simulink model "TRIAD"  (R2017a)
settings: Solver=ode4  StartTime=0.0  StopTime=20000  FixedStep=0.1  RelTol=1e-3  EnableMultiTasking=on
undefined symbols (not defined in the file): mbaseserialmask, RxBuffer
libraries: xpcseriallib x17, vrlib x7, slrtlib x4, sharedtransform x3, sharedutil x2, dspinverses x2, dspmathops x2, simulink x1, dspsigops x1
(part 1 of 3)
settings Model: Creator=yhj  LastModifiedBy=ATLAS
settings SolverCC: EnableConcurrentExecution=on  ConcurrentTasks=on  AutoInsertRateTranBlk=on
settings DataIOCC: SaveFormat=StructureWithTime
settings OptimizationCC: BlockReduction=off  OptimizeBlockIOStorage=off  BufferReuse=off  GlobalBufferReuse=off  ExpressionFolding=off  LocalBlockOutputs=off
settings HardwareCC: ProdBitPerPointer=32  ProdBitPerSizeT=32  ProdBitPerPtrDiffT=32  ProdLargestAtomicFloat=None  ProdWordSize=32  ProdLongLongMode=on  ProdHWDeviceType=Generic->32-bit x86 compatible
settings RTWCC: SystemTargetFile=slrt.tlc  TemplateMakefile=slrt_default_tmf  Description=Simulink Real-Time  RTWCompilerOptimization=on
settings SimulinkRealTimeCC: xPCConcurrentTasks=on

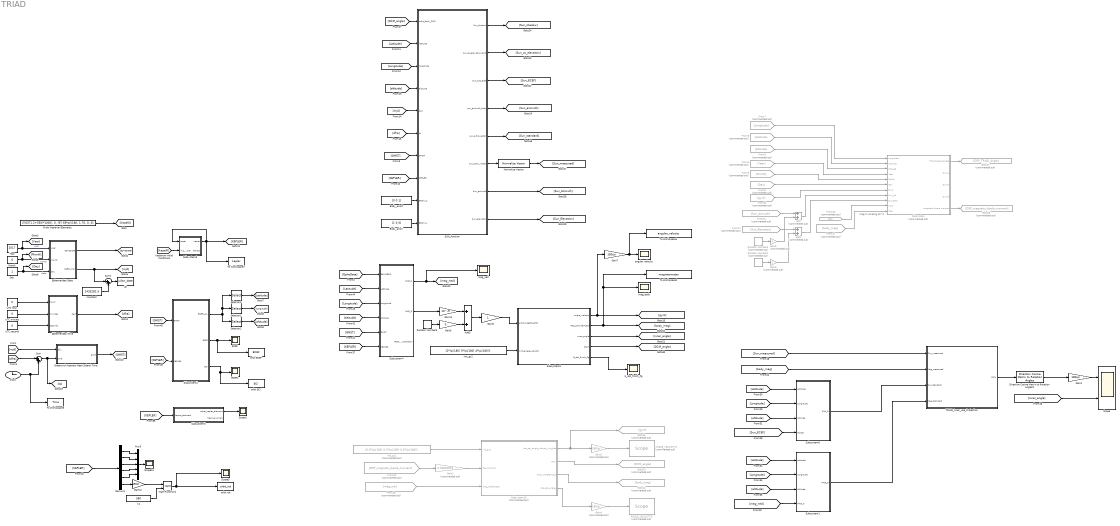
== system TRIAD ==
  note: mag =>scaling 10^3
  ANGLE_VELOCITY2 : slrtlib/Displays and Logging/Scope   Commented=on  scopeno=3  scopetype=Target  autostart=on  viewmode=Numerical  formatstr='%15.6f'  grid=on  ylimits=[-180,180]  nosamples=3  noprepostsamples=0  interleave=10  triggermode=FreeRun  triggersignal=1  trigsignalfromport=off  triggerlevel=0.0  triggerslope=Either  triggerscope=1  triggersample=0  filename=ANGLE2.dat  mode=Lazy  writesize=512  autorestart=off  dynamicfilemode=off  maxwritefilesize=512*1024^2
  ANGLE_VELOCITY3 : slrtlib/Displays and Logging/Scope   Commented=on  scopeno=7  scopetype=Target  autostart=on  viewmode=Numerical  formatstr='%15.6f'  grid=on  ylimits=[-180,180]  nosamples=3  noprepostsamples=0  interleave=10  triggermode=FreeRun  triggersignal=1  trigsignalfromport=off  triggerlevel=0.0  triggerslope=Either  triggerscope=1  triggersample=0  filename=ANGLE2.dat  mode=Lazy  writesize=512  autorestart=off  dynamicfilemode=off  maxwritefilesize=512*1024^2
  Add3 : Sum
  Body_axisX : Constant  Value=[1 0 0]  VectorParams1D=off
  Body_axisZ : Constant  Value=[0 0 1]  VectorParams1D=off
  Clock : Clock
  Day : Constant
  Demux3 : Demux  Outputs=6
  Direction Cosine Matrix to Rotation Angles2 : sharedtransform/Direction Cosine Matrix to Rotation Angles  rotationOrder=ZYX  lim=Default
  ECEF : Scope
  ECEF1 : Scope
  Ephemerides Date : Subsystem
  Ephemerides Time : MATLAB Function  TreatAsAtomicUnit=on
  From17 : From  Commented=on  GotoTag=Sun_Elevation
  From19 : From  Commented=on  GotoTag=mag_orb
  From20 : From  Commented=on  GotoTag=DSP_magnetic_dipole_moment
  From21 : From  Commented=on  GotoTag=gyro
  From23 : From  Commented=on  GotoTag=ts
  From4 : From  Commented=on  GotoTag=Year
  From47 : From  Commented=on  GotoTag=body_mag
  From5 : From  Commented=on  GotoTag=Month
  From51 : From  Commented=on  GotoTag=Sun_Azimuth
  From6 : From  Commented=on  GotoTag=Day
  From7 : From  Commented=on  GotoTag=Longitude
  From8 : From  Commented=on  GotoTag=Latitude
  From9 : From  Commented=on  GotoTag=altitude
  Gain1 : Gain  Gain=180/pi
  Gain11 : Gain  Gain=10^-9
  Gain12 : Gain  Gain=180/pi
  Gain2 : Gain  Commented=on  Gain=0.00000001
  Gain3 : Gain  Commented=on  Gain=180/pi
  Gain4 : Gain  Commented=on  Gain=180/pi
  Gain5 : Gain  Gain=0
  Gain6 : Gain
  Gain7 : Gain  Gain=180/pi
  Gain8 : Gain  Commented=on  Gain=0
  Gain9 : Gain  Commented=on  Gain=0
  Goto12 : Goto  Commented=on  GotoTag=body_mag
  Goto23 : Goto  Commented=on  GotoTag=DCM_angle
  Goto25 : Goto  Commented=on  GotoTag=gyro
  Goto26 : Goto  Commented=on  GotoTag=DSP_magnetic_dipole_moment
  Goto27 : Goto  Commented=on  GotoTag=DSP_TRIAD_Angle
  Greenwich Aparent Mean Sideral Time : MATLAB Function  TreatAsAtomicUnit=on
  JD : ToWorkspace  VariableName=Julian_date  SampleTime=-1
  Math Function1 : Math  Operator=rem  SaturateOnIntegerOverflow=on
  Month : Constant  Value=6
  Mux3 : Mux  Inputs=5
  Normalize Vector : vrlib/Utilities/Normalize Vector  maxzero=0
      settings: SourceProductName=Simulink 3D Animation  SourceProductBaseCode=VR
  Orbit Keplerian Elements : Constant  Value=[((6371.2+550)*1000), 0, (97.69*pi)/180, 1.76, 0, 0]
  Random Number2 : RandomNumber  Commented=on  Variance=0.035^2
  Random Number3 : RandomNumber  Commented=on  Variance=0.035^2
  Random Number9 : RandomNumber  Variance=(3*10^-7)^2
  SUN_function : Subsystem
  Scope : Scope  NumInputPorts=2
  Scope1 : Scope
  Scope24 : Scope
  Scope3 : Scope
  Selector1 : Selector  InputPortWidth=3  IndexOptions=Index vector (dialog)  Indices=[1]  OutputSizes=1
  Selector2 : Selector  InputPortWidth=3  IndexOptions=Index vector (dialog)  Indices=[3]  OutputSizes=1
  Selector3 : Selector  InputPortWidth=3  IndexOptions=Index vector (dialog)  Indices=[2]  OutputSizes=1
  Subsystem : Subsystem  Commented=on
  Subsystem1 : Subsystem
  Subsystem10 : Subsystem  Commented=on
  Subsystem2 : Subsystem
  Subsystem3 : Subsystem
  Subsystem4 : Subsystem
  Subsystem5 : Subsystem
  Subsystem6 : Subsystem
  Subsystem9 : Subsystem
  Sum : Sum  Inputs=|++
  Sum1 : Sum  Inputs=|++
  TRIAD_inner_use_Projection : Subsystem
  To Workspace1 : ToWorkspace  VariableName=angular_velocity  SampleTime=-1
  To Workspace2 : ToWorkspace  VariableName=magnetometer  SampleTime=-1
  To Workspace3 : ToWorkspace  VariableName=Time  SampleTime=-1
  To Workspace7 : ToWorkspace  VariableName=kepler  SampleTime=-1
      settings: Save2DSignal=2-D array (concatenate along first dimension)
  UTC hour : Constant  Value=0
  UTC minute : Constant  Value=0
  UTC second : Constant  Value=0
  Year : Constant  Value=2017
  add : Sum  Commented=on
  add1 : Sum  Commented=on
  angular velocity : Scope
  b_dot_finish_flg : Scope
  constant : Constant  Value=2433282.5
  init_gy1 : Constant  Commented=on  Value=[0.5*(pi/180) 0.5*(pi/180) 0.5*(pi/180)]'
  init_gy2 : Constant  Value=[2*(pi/180) 5*(pi/180) 4*(pi/180)]'
  k1 : Constant  Value=360
  mag_body : Scope
  mag_ned : Scope
  orbit ECEF : ToWorkspace  VariableName=ECEF  SampleTime=-1
      settings: Save2DSignal=2-D array (concatenate along first dimension)
  orbit ECI : ToWorkspace  VariableName=ECI  SampleTime=-1
      settings: Save2DSignal=2-D array (concatenate along first dimension)
  orbit rot : ToWorkspace  VariableName=orbit_rot  SampleTime=-1
  wires:
  Gain6/1 -> Subsystem9/1(orbit_mag[GAUSS])
  Subsystem9/1(angle_velocity) -> Gain7/1, [gyro]
  Subsystem10/3(body_mag[GAUSS]) -> Goto12/1
  Subsystem10/2(dcm) -> Goto23/1
  Subsystem9/3(inner_angle) -> [inner_angle]
  SUN_function/8(Sun_elevation) -> [Sun_Elevation]
  SUN_function/1(Sun_shadow) -> [Sun_shadow]
  SUN_function/2(sun_co_elevation_body) -> [Sun_co_elevation]
  UTC minute/1 -> Ephemerides Time/2(minutes)
  Subsystem/5(magnetic dipole moment) -> Goto26/1
  [KEPLER] -> Subsystem2/2(KEPLER)
  From47/1 -> Subsystem/11(Mag)
  Subsystem6/1(SUN_O) -> TRIAD_inner_use_Projection/3(Sun_standard)
  [KEPLER] -> Subsystem4/6(KEPLER)
  SUN_function/7(Sun_azimuth) -> [Sun_Azimuth]
  Subsystem3/1(other_kepler_element) -> Scope1/1
  [dfra] -> Sum/1
  Ephemerides Time/1(dayf) -> [dfra]
  Selector1/1 -> [Longitude]
  Greenwich Aparent Mean Sideral Time/1(gwst) -> [GMST]
  UTC second/1 -> Ephemerides Time/3(seconds)
  Day/1 -> [Day], Ephemerides Date/3(day)  "date"
  [KEPLER] -> SUN_function/8(KEPLER)
  Selector3/1 -> [Latitude]
  From7/1 -> Subsystem/1(Longitude)
  Sum/1 -> [ts], Greenwich Aparent Mean Sideral Time/2(time)
  Ephemerides Date/2(CNES_mdj) -> Sum1/1, [mjd]
  [Longitude] -> Subsystem6/2(Longitude)
  Sum1/1 -> JD/1
  Year/1 -> Ephemerides Date/1(year), [Year]  "year"
  [KEPLER] -> Subsystem3/1(kepler_element)
  Clock/1 -> To Workspace3/1, Sum/2
  UTC hour/1 -> Ephemerides Time/1(hours)
  TRIAD_inner_use_Projection/1(DCM) -> Direction Cosine Matrix to Rotation Angles2/1
  Ephemerides Date/1(EpheDate) -> [EpheDate]
  Orbit Keplerian Elements/1 -> [kepel0]
  SUN_function/4(sun_azimuth_body) -> [Sun_azimuth]
  Normalize Vector/1 -> [Sun_measured]
  [dfra] -> SUN_function/6(ts)
  [altitude] -> Subsystem1/3(Altitude)
  [EpheDate] -> Subsystem4/1(EPHMERIS)
  [mag_ned] -> Subsystem1/4(MAG_N)
  [Sun_ECEF] -> Subsystem6/4(SUN_E)
  Subsystem2/1(ECEF_LLA) -> Selector3/1, Selector1/1, Selector2/1
  [Latitude] -> Subsystem4/2(Latitude)
  [body_mag] -> TRIAD_inner_use_Projection/2(Mag_measured)
  [Longitude] -> Subsystem1/2(Longitude)
  [Longitude] -> SUN_function/3(longitude)
  Add3/1 -> Gain6/1
  Month/1 -> [Month], Ephemerides Date/2(month)  "month"
  From4/1 -> Subsystem/4(Year)
  From5/1 -> Subsystem/5(Month)
  [Latitude] -> Subsystem1/1(Latitude)
  constant/1 -> Sum1/2
  add1/1 -> Subsystem/9(Sun_Elev)
  Subsystem1/1(MAG_O) -> TRIAD_inner_use_Projection/4(Mag_standard)
  Subsystem5/1(kepler) -> To Workspace7/1, [KEPLER], Subsystem5/1(kepel)
  [Latitude] -> Subsystem6/1(Latitude)
  Random Number3/1 -> Gain8/1
  add/1 -> Subsystem/8(Sun_Azi)
  From8/1 -> Subsystem/2(Latitude)
  [GMST] -> Subsystem4/5(GMST)
  [altitude] -> Subsystem4/4(Altitude)
  From23/1 -> Subsystem/10(HMS)
  Gain2/1 -> Subsystem10/2(dsp_moment)
  From21/1 -> Subsystem/7(Gyro)
  SUN_function/3(Sun_pos_ecef) -> [Sun_ECEF]
  init_gy1/1 -> Subsystem10/1(init_gyro)
  From51/1 -> add/1
  Random Number9/1 -> Gain5/1
  Random Number2/1 -> Gain9/1
  Gain3/1 -> ANGLE_VELOCITY2/1
  From9/1 -> Subsystem/3(Altitude)
  Subsystem4/1(MAG_N) -> mag_ned/1, [mag_ned]
  [mjd] -> SUN_function/5(djm)
  [Longitude] -> Subsystem4/3(Longitude)
  [altitude] -> Subsystem6/3(Altitude)
  [Latitude] -> SUN_function/2(latitude)
  SUN_function/6(sun_body_vector) -> Normalize Vector/1
  Gain11/1 -> Add3/1
  [Sun_measured] -> TRIAD_inner_use_Projection/1(Sun_measured)
  [DCM_angle] -> SUN_function/1(orbit_body_DCM)
  [mjd] -> Greenwich Aparent Mean Sideral Time/1(diju)
  Body_axisX/1 -> SUN_function/10(BODY_X)
  Subsystem10/1(dsp_cal_angle_velocity_wrt_bdot) -> Goto25/1, Gain3/1
  Subsystem/1(TRAID_result_angle) -> Goto27/1
  SUN_function/5(sun_orbit_vector) -> [Sun_standard]
  [GMST] -> SUN_function/7(GMST)
  [kepel0] -> Subsystem5/2(init_kepler)
  From6/1 -> Subsystem/6(Day)
  From19/1 -> Subsystem10/3(mag_orb[GAUSS])
  Subsystem4/2(MAG_O) -> Gain11/1
  From17/1 -> add1/1
  From20/1 -> Gain2/1
  [altitude] -> SUN_function/4(altitude)
  Body_axisZ/1 -> SUN_function/9(BODY_Z)
  Selector2/1 -> [altitude]
  [GMST] -> Subsystem2/1(GMST)
  Direction Cosine Matrix to Rotation Angles2/1 -> Gain1/1
  Subsystem10/4(dsp_cal_angle_) -> Gain4/1
  Gain4/1 -> ANGLE_VELOCITY3/1
  Gain5/1 -> Add3/2
  Gain8/1 -> add/2
  Gain9/1 -> add1/2
  init_gy2/1 -> Subsystem9/2(iinit_angle_velocity)
  Subsystem9/4(DCM) -> [DCM_angle]
  Subsystem9/2(Mag_body[GAUSS]) -> mag_body/1, To Workspace2/1, [body_mag]
  Gain1/1 -> Scope/1
  [inner_angle] -> Scope/2
  Gain7/1 -> To Workspace1/1, angular velocity/1
  Demux3/3 -> Mux3/3
  Demux3/1 -> Mux3/1
  Math Function1/1 -> Scope3/1, orbit rot/1
  Mux3/1 -> Scope24/1
  Demux3/4 -> Mux3/4
  Demux3/2 -> Mux3/2
  Demux3/6 -> Gain12/1
  Gain12/1 -> Math Function1/1
  k1/1 -> Math Function1/2
  Demux3/5 -> Mux3/5
  [KEPLER] -> Demux3/1
  Subsystem2/2(ECEF) -> ECEF/1, orbit ECEF/1
  Subsystem2/3(ECI) -> ECEF1/1, orbit ECI/1
  Subsystem9/5(B_dot_finish_flg) -> b_dot_finish_flg/1

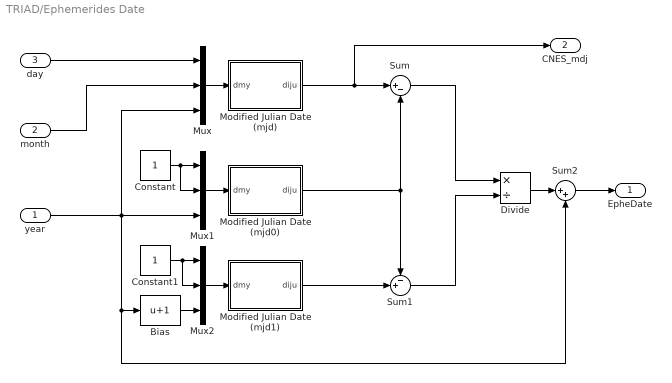
== system TRIAD/Ephemerides Date ==
  year : Inport
  month : Inport  Port=2
  day : Inport  Port=3
  Bias : Bias  Bias=1
  Constant : Constant
  Constant1 : Constant
  Divide : Product  Inputs=*/
  Modified Julian Date (mjd) : MATLAB Function  TreatAsAtomicUnit=on
  Modified Julian Date (mjd0) : MATLAB Function  TreatAsAtomicUnit=on
  Modified Julian Date (mjd1) : MATLAB Function  TreatAsAtomicUnit=on
  Mux : Mux  Inputs=3
  Mux1 : Mux  Inputs=3
  Mux2 : Mux  Inputs=3
  Sum : Sum  Inputs=|+-
  Sum1 : Sum  Inputs=-+|
  Sum2 : Sum  Inputs=|++
  EpheDate : Outport
  CNES_mdj : Outport  Port=2
  wires:
  Sum1/1 -> Divide/2
  Modified Julian Date (mjd1)/1(diju) -> Sum1/2
  month/1 -> Mux/2
  year/1 -> Mux1/3, Mux/3, Bias/1, Sum2/2
  Mux1/1 -> Modified Julian Date (mjd0)/1(dmy)
  day/1 -> Mux/1
  Mux/1 -> Modified Julian Date (mjd)/1(dmy)
  Mux2/1 -> Modified Julian Date (mjd1)/1(dmy)
  Bias/1 -> Mux2/3
  Modified Julian Date (mjd)/1(diju) -> CNES_mdj/1, Sum/1
  Constant1/1 -> Mux2/2, Mux2/1
  Sum/1 -> Divide/1
  Constant/1 -> Mux1/2, Mux1/1
  Modified Julian Date (mjd0)/1(diju) -> Sum1/1, Sum/2
  Divide/1 -> Sum2/1
  Sum2/1 -> EpheDate/1

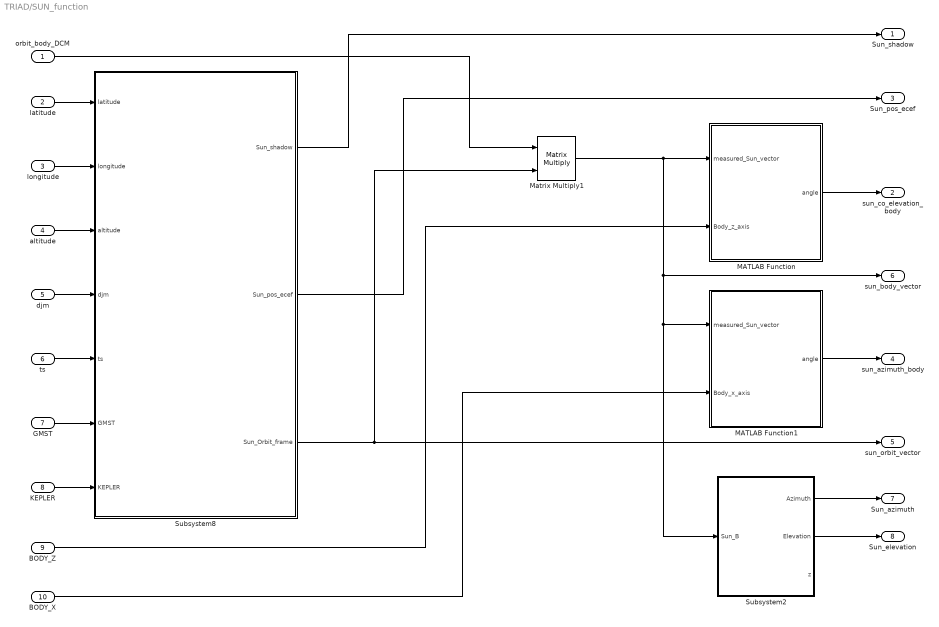
== system TRIAD/SUN_function ==
  orbit_body_DCM : Inport
  latitude : Inport  Port=2
  longitude : Inport  Port=3
  altitude : Inport  Port=4
  djm : Inport  Port=5
  ts : Inport  Port=6
  GMST : Inport  Port=7
  KEPLER : Inport  Port=8
  BODY_Z : Inport  Port=9
  BODY_X : Inport  Port=10
  MATLAB Function : MATLAB Function  TreatAsAtomicUnit=on
  MATLAB Function1 : MATLAB Function  TreatAsAtomicUnit=on
  Matrix Multiply1 : Product  Multiplication=Matrix(*)
  Subsystem2 : Subsystem
  Subsystem8 : Subsystem
  Sun_shadow : Outport
  sun_co_elevation_body : Outport  Port=2
  Sun_pos_ecef : Outport  Port=3
  sun_azimuth_body : Outport  Port=4
  sun_orbit_vector : Outport  Port=5
  sun_body_vector : Outport  Port=6
  Sun_azimuth : Outport  Port=7
  Sun_elevation : Outport  Port=8
  wires:
  Subsystem8/1(Sun_shadow) -> Sun_shadow/1
  Matrix Multiply1/1 -> sun_body_vector/1, Subsystem2/1(Sun_B), MATLAB Function1/1(measured_Sun_vector), MATLAB Function/1(measured_Sun_vector)
  MATLAB Function1/1(angle) -> sun_azimuth_body/1
  BODY_Z/1 -> MATLAB Function/2(Body_z_axis)
  GMST/1 -> Subsystem8/6(GMST)
  latitude/1 -> Subsystem8/1(latitude)
  longitude/1 -> Subsystem8/2(longitude)
  djm/1 -> Subsystem8/4(djm)
  ts/1 -> Subsystem8/5(ts)
  KEPLER/1 -> Subsystem8/7(KEPLER)
  altitude/1 -> Subsystem8/3(altitude)
  MATLAB Function/1(angle) -> sun_co_elevation_body/1
  orbit_body_DCM/1 -> Matrix Multiply1/1
  Subsystem8/2(Sun_pos_ecef) -> Sun_pos_ecef/1
  BODY_X/1 -> MATLAB Function1/2(Body_x_axis)
  Subsystem2/1(Azimuth) -> Sun_azimuth/1
  Subsystem2/2(Elevation) -> Sun_elevation/1
  Subsystem8/3(Sun_Orbit_frame) -> Matrix Multiply1/2, sun_orbit_vector/1

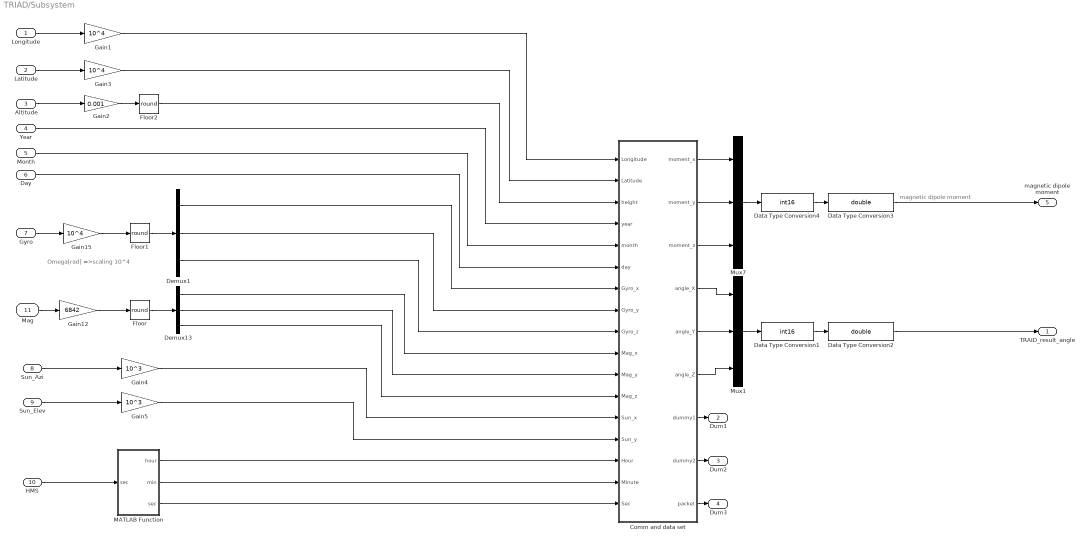
== system TRIAD/Subsystem ==
  note: Omega[rad] =>scaling 10^4
  note: magnetic dipole moment
  Longitude : Inport
  Latitude : Inport  Port=2
  Altitude : Inport  Port=3
  Year : Inport  Port=4
  Month : Inport  Port=5
  Day : Inport  Port=6
  Gyro : Inport  Port=7
  Sun_Azi : Inport  Port=8
  Sun_Elev : Inport  Port=9
  HMS : Inport  Port=10
  Mag : Inport  Port=11
  Comm and data set : Subsystem
  Data Type Conversion1 : DataTypeConversion  OutDataTypeStr=int16
  Data Type Conversion2 : DataTypeConversion  OutDataTypeStr=double
  Data Type Conversion3 : DataTypeConversion  OutDataTypeStr=double
  Data Type Conversion4 : DataTypeConversion  OutDataTypeStr=int16
  Demux1 : Demux  Outputs=3
  Demux13 : Demux  Outputs=3
  Floor : Rounding  Operator=round
  Floor1 : Rounding  Operator=round
  Floor2 : Rounding  Operator=round
  Gain1 : Gain  Gain=10^4
  Gain12 : Gain  Gain=6842
  Gain15 : Gain  Gain=10^4
  Gain2 : Gain  Gain=0.001
  Gain3 : Gain  Gain=10^4
  Gain4 : Gain  Gain=10^3
  Gain5 : Gain  Gain=10^3
  MATLAB Function : MATLAB Function  TreatAsAtomicUnit=on
  Mux1 : Mux  Inputs=3
  Mux7 : Mux  Inputs=3
  TRAID_result_angle : Outport
  Dum1 : Outport  Port=2
  Dum2 : Outport  Port=3
  Dum3 : Outport  Port=4
  magnetic dipole moment : Outport  Port=5
  wires:
  Data Type Conversion4/1 -> Data Type Conversion3/1
  Gain12/1 -> Floor/1
  Longitude/1 -> Gain1/1
  Demux13/2 -> Comm and data set/11(Mag_y)
  Altitude/1 -> Gain2/1
  Latitude/1 -> Gain3/1
  Demux13/3 -> Comm and data set/12(Mag_z)
  Comm and data set/1(moment_x) -> Mux7/1
  Comm and data set/2(moment_y) -> Mux7/2
  Comm and data set/3(moment_z) -> Mux7/3
  Demux13/1 -> Comm and data set/10(Mag_x)
  Mux7/1 -> Data Type Conversion4/1
  Floor/1 -> Demux13/1
  Year/1 -> Comm and data set/4(year)
  Month/1 -> Comm and data set/5(month)
  Day/1 -> Comm and data set/6(day)
  Gyro/1 -> Gain15/1
  Gain1/1 -> Comm and data set/1(Longitude)
  Gain3/1 -> Comm and data set/2(Latitude)
  Demux1/1 -> Comm and data set/7(Gyro_x)
  Demux1/2 -> Comm and data set/8(Gyro_y)
  Demux1/3 -> Comm and data set/9(Gyro_z)
  Gain15/1 -> Floor1/1
  Comm and data set/4(angle_X) -> Mux1/1
  Comm and data set/5(angle_Y) -> Mux1/2
  Comm and data set/6(angle_Z) -> Mux1/3
  Mux1/1 -> Data Type Conversion1/1
  Data Type Conversion1/1 -> Data Type Conversion2/1
  Floor1/1 -> Demux1/1
  MATLAB Function/1(hour) -> Comm and data set/15(Hour)
  HMS/1 -> MATLAB Function/1("sec ")
  Sun_Azi/1 -> Gain4/1
  Sun_Elev/1 -> Gain5/1
  MATLAB Function/2(min) -> Comm and data set/16(Minute)
  MATLAB Function/3(sec) -> Comm and data set/17(Sec)
  Data Type Conversion3/1 -> magnetic dipole moment/1
  Floor2/1 -> Comm and data set/3(height)
  Gain2/1 -> Floor2/1
  Data Type Conversion2/1 -> TRAID_result_angle/1
  Comm and data set/7(dummy1) -> Dum1/1
  Mag/1 -> Gain12/1
  Comm and data set/8(dummy2) -> Dum2/1
  Comm and data set/9(packet) -> Dum3/1
  Gain5/1 -> Comm and data set/14(Sun_y)
  Gain4/1 -> Comm and data set/13(Sun_x)

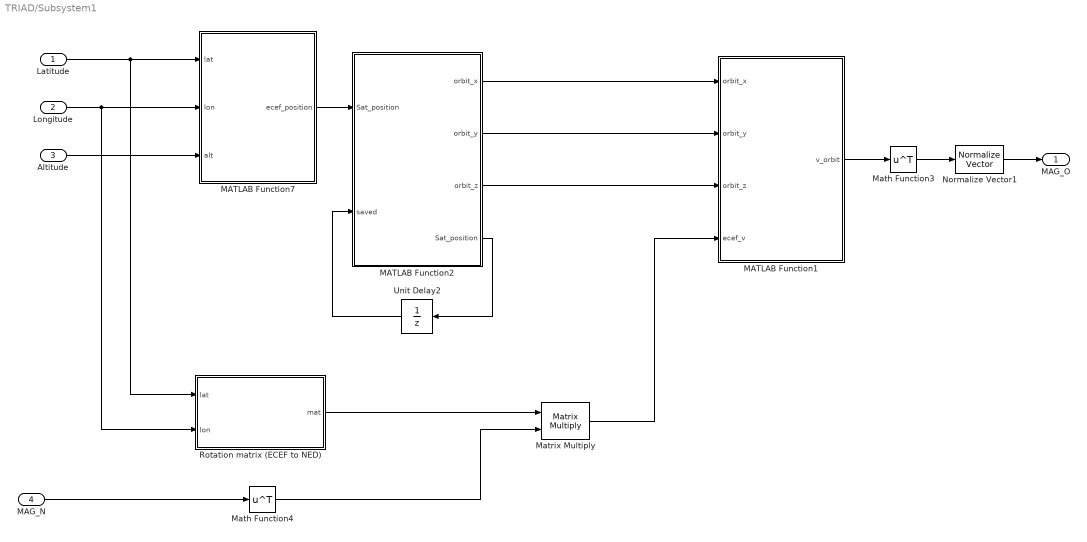
== system TRIAD/Subsystem1 ==
  Latitude : Inport
  Longitude : Inport  Port=2
  Altitude : Inport  Port=3
  MAG_N : Inport  Port=4
  MATLAB Function1 : MATLAB Function  TreatAsAtomicUnit=on
  MATLAB Function2 : MATLAB Function  TreatAsAtomicUnit=on
  MATLAB Function7 : MATLAB Function  TreatAsAtomicUnit=on
  Math Function3 : Math  Operator=transpose  SaturateOnIntegerOverflow=on
  Math Function4 : Math  Operator=transpose  SaturateOnIntegerOverflow=on
  Matrix Multiply : Product  Multiplication=Matrix(*)
  Normalize Vector1 : vrlib/Utilities/Normalize Vector  maxzero=0
      settings: SourceProductName=Simulink 3D Animation  SourceProductBaseCode=VR
  Rotation matrix (ECEF to NED) : MATLAB Function  TreatAsAtomicUnit=on
  Unit Delay2 : UnitDelay  InitialCondition=[0;0;0]  SampleTime=0.1
  MAG_O : Outport
  wires:
  MATLAB Function1/1(v_orbit) -> Math Function3/1
  Rotation matrix (ECEF to NED)/1(mat) -> Matrix Multiply/1
  MAG_N/1 -> Math Function4/1
  Math Function3/1 -> Normalize Vector1/1
  MATLAB Function2/2(orbit_y) -> MATLAB Function1/2(orbit_y)
  Math Function4/1 -> Matrix Multiply/2
  Matrix Multiply/1 -> MATLAB Function1/4(ecef_v)
  MATLAB Function2/1(orbit_x) -> MATLAB Function1/1(orbit_x)
  Altitude/1 -> MATLAB Function7/3(alt)
  Latitude/1 -> Rotation matrix (ECEF to NED)/1(lat), MATLAB Function7/1(lat)
  Longitude/1 -> Rotation matrix (ECEF to NED)/2(lon), MATLAB Function7/2(lon)
  MATLAB Function2/4(Sat_position) -> Unit Delay2/1
  MATLAB Function2/3(orbit_z) -> MATLAB Function1/3(orbit_z)
  Unit Delay2/1 -> MATLAB Function2/2(saved)
  Normalize Vector1/1 -> MAG_O/1
  MATLAB Function7/1(ecef_position) -> MATLAB Function2/1("Sat_position ")

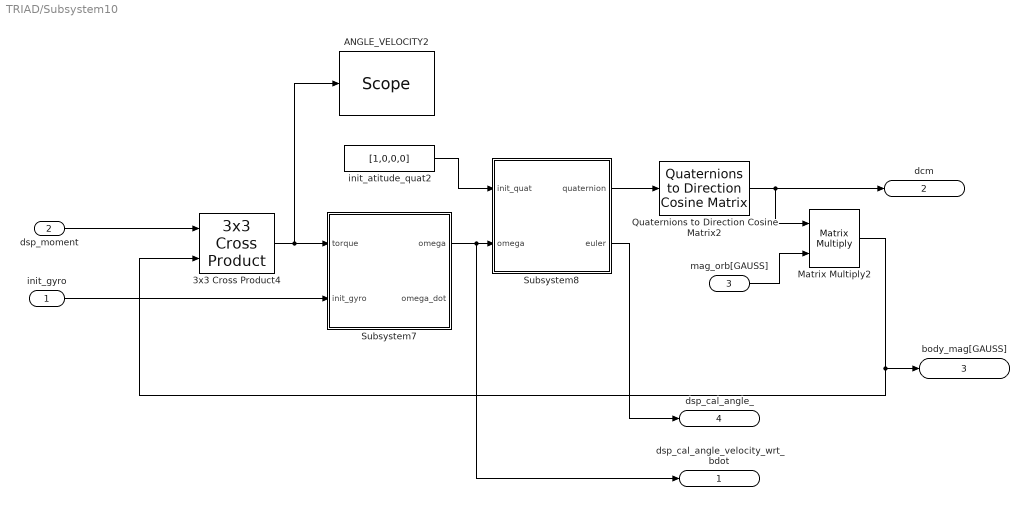
== system TRIAD/Subsystem10 ==
  init_gyro : Inport
  dsp_moment : Inport  Port=2
  mag_orb[GAUSS] : Inport  Port=3
  3x3 Cross Product4 : sharedutil/3x3 Cross Product
      settings: SourceProductName=The database C:\Users\yhj\AppData\Roaming\MathWorks\MATLAB\R2017a\slblocks_master.db is locked, or a table in the database is locked. (database is locked)
  ANGLE_VELOCITY2 : slrtlib/Displays and Logging/Scope   scopeno=5  scopetype=Target  autostart=on  viewmode=Numerical  formatstr='%15.6f'  grid=on  ylimits=[-180,180]  nosamples=3  noprepostsamples=0  interleave=10  triggermode=FreeRun  triggersignal=1  trigsignalfromport=off  triggerlevel=0.0  triggerslope=Either  triggerscope=1  triggersample=0  filename=ANGLE2.dat  mode=Lazy  writesize=512  autorestart=off  dynamicfilemode=off  maxwritefilesize=512*1024^2
  Matrix Multiply2 : Product  Multiplication=Matrix(*)
  Quaternions to Direction Cosine Matrix2 : sharedtransform/Quaternions to  Direction Cosine Matrix
  Subsystem7 : Subsystem
  Subsystem8 : Subsystem
  init_atitude_quat2 : Constant  Value=[1,0,0,0]
  dsp_cal_angle_velocity_wrt_bdot : Outport
  dcm : Outport  Port=2
  body_mag[GAUSS] : Outport  Port=3
  dsp_cal_angle_ : Outport  Port=4
  wires:
  mag_orb[GAUSS]/1 -> Matrix Multiply2/2
  init_gyro/1 -> Subsystem7/2(init_gyro)
  Subsystem7/1(omega) -> Subsystem8/2(omega), dsp_cal_angle_velocity_wrt_bdot/1
  Subsystem8/1(quaternion) -> Quaternions to Direction Cosine Matrix2/1
  Quaternions to Direction Cosine Matrix2/1 -> Matrix Multiply2/1, dcm/1
  3x3 Cross Product4/1 -> ANGLE_VELOCITY2/1, Subsystem7/1(torque)
  init_atitude_quat2/1 -> Subsystem8/1(init_quat)
  Matrix Multiply2/1 -> body_mag[GAUSS]/1, 3x3 Cross Product4/2
  dsp_moment/1 -> 3x3 Cross Product4/1
  Subsystem8/2(euler) -> dsp_cal_angle_/1

== system TRIAD/Subsystem2 ==
  note: alt = sphe(3)/1000
      | elong = sphe(1)
      | colat = pi/2-sphe(2)
  GMST : Inport
  KEPLER : Inport  Port=2
  Convert Keplerian parameters to states : MATLAB Function  TreatAsAtomicUnit=on
  Convert Terrestrial Geocentric to Speherical coordinates ECEF2LLA : MATLAB Function  TreatAsAtomicUnit=on
  "ECI to ECEF " : MATLAB Function  TreatAsAtomicUnit=on
  ECEF_LLA : Outport
  ECEF : Outport  Port=2
  ECI : Outport  Port=3
  wires:
  "ECI to ECEF "/1(xterrestrial) -> ECEF/1, Convert Terrestrial Geocentric to Speherical coordinates ECEF2LLA/1(geoc)  "geoc"
  Convert Terrestrial Geocentric to Speherical coordinates ECEF2LLA/1(spherical) -> ECEF_LLA/1
  Convert Keplerian parameters to states/1(statvec) -> "ECI to ECEF "/2(xi), ECI/1
  GMST/1 -> "ECI to ECEF "/1(tesig)
  KEPLER/1 -> Convert Keplerian parameters to states/1(kepel)

== system TRIAD/Subsystem3 ==
  kepler_element : Inport
  Demux3 : Demux  Outputs=6
  Gain1 : Gain  Gain=180/pi
  Math Function1 : Math  Operator=rem  SaturateOnIntegerOverflow=on
  Mux3 : Mux  Inputs=5
  k1 : Constant  Value=360
  other_kepler_element : Outport
  Mean_anomaly : Outport  Port=2
  wires:
  kepler_element/1 -> Demux3/1
  Demux3/2 -> Mux3/2
  k1/1 -> Math Function1/2
  Demux3/1 -> Mux3/1
  Math Function1/1 -> Mean_anomaly/1
  Demux3/3 -> Mux3/3
  Mux3/1 -> other_kepler_element/1
  Demux3/6 -> Gain1/1
  Demux3/4 -> Mux3/4
  Gain1/1 -> Math Function1/1
  Demux3/5 -> Mux3/5

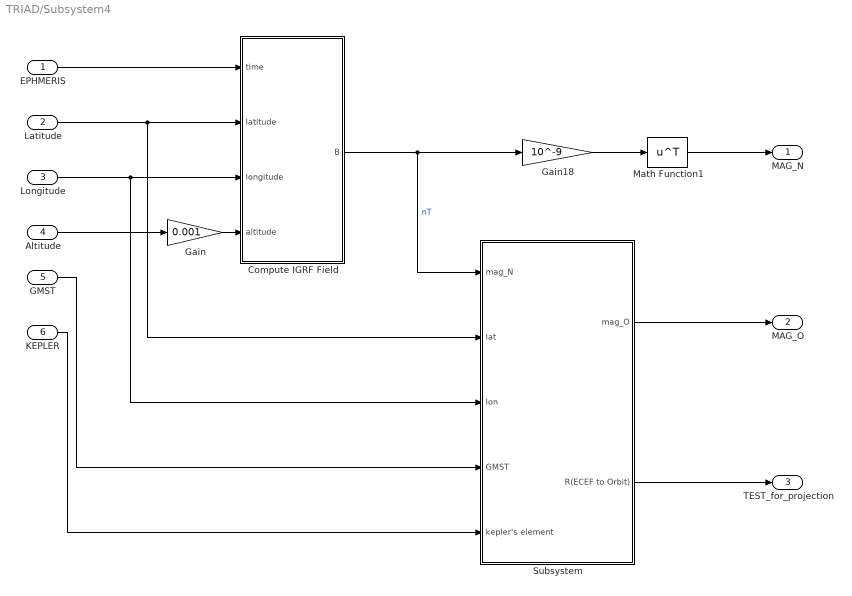
== system TRIAD/Subsystem4 ==
  EPHMERIS : Inport
  Latitude : Inport  Port=2
  Longitude : Inport  Port=3
  Altitude : Inport  Port=4
  GMST : Inport  Port=5
  KEPLER : Inport  Port=6
  Compute IGRF Field : MATLAB Function  TreatAsAtomicUnit=on
  Gain : Gain  Gain=0.001
  Gain18 : Gain  Gain=10^-9
  Math Function1 : Math  Operator=transpose  SaturateOnIntegerOverflow=on
  Subsystem : Subsystem
  MAG_N : Outport
  MAG_O : Outport  Port=2
  TEST_for_projection : Outport  Port=3
  wires:
  Compute IGRF Field/1(B) -> Gain18/1, Subsystem/1(mag_N)  "nT"
  Subsystem/1(mag_O) -> MAG_O/1
  Gain/1 -> Compute IGRF Field/4(altitude)
  EPHMERIS/1 -> Compute IGRF Field/1(time)
  Gain18/1 -> Math Function1/1
  Latitude/1 -> Subsystem/2(lat), Compute IGRF Field/2(latitude)
  Longitude/1 -> Subsystem/3(lon), Compute IGRF Field/3(longitude)
  GMST/1 -> Subsystem/4(GMST)
  Subsystem/2(R(ECEF to Orbit)) -> TEST_for_projection/1
  Math Function1/1 -> MAG_N/1
  Altitude/1 -> Gain/1
  KEPLER/1 -> Subsystem/5(kepler's element)

== system TRIAD/Subsystem5 ==
  kepel : Inport
  init_kepler : Inport  Port=2
  Integrator : Integrator  InitialConditionSource=external
  Keplerian Differential Equation : MATLAB Function  TreatAsAtomicUnit=on
  kepler : Outport
  delkep : Outport  Port=2
  wires:
  Integrator/1 -> kepler/1  "kepel"
  Keplerian Differential Equation/1(deltakep) -> delkep/1, Integrator/1
  init_kepler/1 -> Integrator/2
  kepel/1 -> Keplerian Differential Equation/1(kepel)

== system TRIAD/Subsystem6 ==
  Latitude : Inport
  Longitude : Inport  Port=2
  Altitude : Inport  Port=3
  SUN_E : Inport  Port=4
  MATLAB Function3 : MATLAB Function  TreatAsAtomicUnit=on
  MATLAB Function4 : MATLAB Function  TreatAsAtomicUnit=on
  MATLAB Function5 : MATLAB Function  TreatAsAtomicUnit=on
  MATLAB Function6 : MATLAB Function  TreatAsAtomicUnit=on
  Math Function2 : Math  Operator=transpose  SaturateOnIntegerOverflow=on
  Normalize Vector2 : vrlib/Utilities/Normalize Vector  maxzero=0
      settings: SourceProductName=Simulink 3D Animation  SourceProductBaseCode=VR
  Unit Delay1 : UnitDelay  InitialCondition=[0;0;0]  SampleTime=0.1
  SUN_O : Outport
  wires:
  MATLAB Function5/1(ecef_position) -> MATLAB Function4/1("Sat_position ")
  Altitude/1 -> MATLAB Function5/3(alt)
  Longitude/1 -> MATLAB Function5/2(lon)
  MATLAB Function4/4(Sat_position) -> Unit Delay1/1
  Unit Delay1/1 -> MATLAB Function4/2(saved)
  MATLAB Function4/1(orbit_x) -> MATLAB Function6/1(orbit_x)
  MATLAB Function4/2(orbit_y) -> MATLAB Function6/2(orbit_y)
  MATLAB Function4/3(orbit_z) -> MATLAB Function6/3(orbit_z)
  MATLAB Function6/1(v_orbit) -> Math Function2/1
  MATLAB Function3/1(y) -> MATLAB Function6/4(ecef_v)
  SUN_E/1 -> MATLAB Function3/1(u)
  Math Function2/1 -> Normalize Vector2/1
  Latitude/1 -> MATLAB Function5/1(lat)
  Normalize Vector2/1 -> SUN_O/1

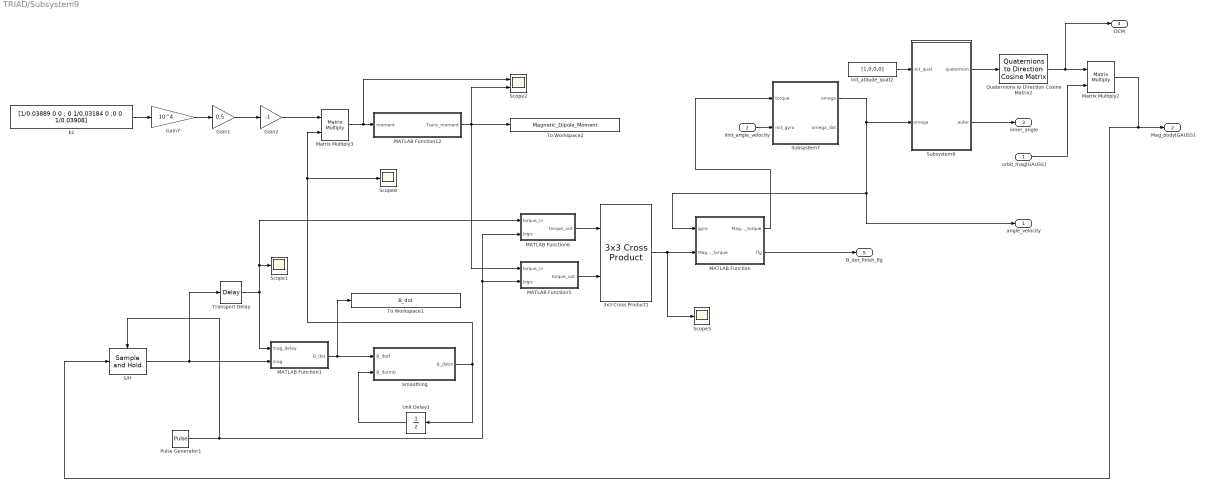
== system TRIAD/Subsystem9 ==
  orbit_mag[GAUSS] : Inport
  iinit_angle_velocity : Inport  Port=2
  3x3 Cross Product1 : sharedutil/3x3 Cross Product
      settings: SourceProductName=The database C:\Users\yhj\AppData\Roaming\MathWorks\MATLAB\R2017a\slblocks_master.db is locked, or a table in the database is locked. (database is locked)
  Gain1 : Gain  Gain=0.5
  Gain2 : Gain  Gain=-1
  Gain7 : Gain  Gain=10^4
  MATLAB Function : MATLAB Function  TreatAsAtomicUnit=on
  MATLAB Function1 : MATLAB Function  TreatAsAtomicUnit=on
  MATLAB Function12 : MATLAB Function  TreatAsAtomicUnit=on
  MATLAB Function5 : MATLAB Function  TreatAsAtomicUnit=on
  MATLAB Function6 : MATLAB Function  TreatAsAtomicUnit=on
  Matrix Multiply2 : Product  Multiplication=Matrix(*)
  Matrix Multiply3 : Product  Multiplication=Matrix(*)
  Pulse Generator1 : DiscretePulseGenerator  PulseType=Time based  Period=1  PulseWidth=50
  Quaternions to Direction Cosine Matrix2 : sharedtransform/Quaternions to  Direction Cosine Matrix
  S/H : dspsigops/Sample and Hold  trig=Rising edge  initCond=0  latchinput=off
  Scope1 : Scope
  Scope2 : Scope  NumInputPorts=2
  Scope3 : Scope
  Scope8 : Scope
  Smoothing : MATLAB Function  TreatAsAtomicUnit=on
  Subsystem7 : Subsystem
  Subsystem8 : Subsystem
  To Workspace1 : ToWorkspace  VariableName=B_dot  SampleTime=-1
  To Workspace2 : ToWorkspace  VariableName=Magnetic_Dipole_Moment  SampleTime=-1
  Transport Delay : TransportDelay
  Unit Delay1 : UnitDelay  InitialCondition=[0;0;0]
  init_atitude_quat2 : Constant  Value=[1,0,0,0]
  k2 : Constant  Value=[1/0.03889 0 0 ; 0 1/0.03184 0 ;0 0 1/0.03908]  VectorParams1D=off
  angle_velocity : Outport
  Mag_body[GAUSS] : Outport  Port=2
  inner_angle : Outport  Port=3
  DCM : Outport  Port=4
  B_dot_finish_flg : Outport  Port=5
  wires:
  Subsystem8/2(euler) -> inner_angle/1
  Smoothing/1(B_dotm) -> Unit Delay1/1, Matrix Multiply3/2, Scope8/1
  Gain2/1 -> Matrix Multiply3/1
  Subsystem8/1(quaternion) -> Quaternions to Direction Cosine Matrix2/1
  Subsystem7/1(omega) -> angle_velocity/1, MATLAB Function/1(gyro), Subsystem8/2(omega)
  orbit_mag[GAUSS]/1 -> Matrix Multiply2/2
  Matrix Multiply2/1 -> S/H/1, Mag_body[GAUSS]/1
  init_atitude_quat2/1 -> Subsystem8/1(init_quat)
  Quaternions to Direction Cosine Matrix2/1 -> DCM/1, Matrix Multiply2/1
  iinit_angle_velocity/1 -> Subsystem7/2(init_gyro)
  k2/1 -> Gain7/1
  Gain7/1 -> Gain1/1
  MATLAB Function1/1(B_dot) -> To Workspace1/1, Smoothing/1(B_dotf)
  Pulse Generator1/1 -> S/H/Trigger, MATLAB Function5/2(logic), MATLAB Function6/2(logic)
  Unit Delay1/1 -> Smoothing/2(B_dotmb)
  MATLAB Function12/1(Trans_moment) -> To Workspace2/1, MATLAB Function5/1(torque_in), Scope2/2
  MATLAB Function6/1(torque_out) -> 3x3 Cross Product1/1
  MATLAB Function5/1(torque_out) -> 3x3 Cross Product1/2
  S/H/1 -> Transport Delay/1, MATLAB Function1/2(mag)
  Transport Delay/1 -> MATLAB Function6/1(torque_in), Scope1/1, MATLAB Function1/1(mag_delay)
  Gain1/1 -> Gain2/1
  Matrix Multiply3/1 -> Scope2/1, MATLAB Function12/1(moment)
  MATLAB Function/2(flg) -> B_dot_finish_flg/1
  3x3 Cross Product1/1 -> Scope3/1, MATLAB Function/2("Magnetic_torque ")
  MATLAB Function/1(Magnetic_torque) -> Subsystem7/1(torque)

== system TRIAD/TRIAD_inner_use_Projection ==
  Sun_measured : Inport
  Mag_measured : Inport  Port=2
  Sun_standard : Inport  Port=3
  Mag_standard : Inport  Port=4
  BODY_TRIAD : MATLAB Function  TreatAsAtomicUnit=on
  Standard_TRIAD : MATLAB Function  TreatAsAtomicUnit=on
  TIRAD_STA_BODY : MATLAB Function  TreatAsAtomicUnit=on
  DCM : Outport
  wires:
  Standard_TRIAD/1(c_triad) -> TIRAD_STA_BODY/2(mat2)
  BODY_TRIAD/1(c_triad) -> TIRAD_STA_BODY/1(mat1)
  Sun_measured/1 -> BODY_TRIAD/1(v)
  Sun_standard/1 -> Standard_TRIAD/1(v)
  TIRAD_STA_BODY/1(c_triad) -> DCM/1
  Mag_standard/1 -> Standard_TRIAD/2(w)
  Mag_measured/1 -> BODY_TRIAD/2(w)

== system TRIAD/SUN_function/Subsystem2 ==
  Sun_B : Inport
  MATLAB Function8 : MATLAB Function  TreatAsAtomicUnit=on
  MATLAB Function9 : MATLAB Function  TreatAsAtomicUnit=on
  Normalize Vector17 : vrlib/Utilities/Normalize Vector  maxzero=0
      settings: SourceProductName=Simulink 3D Animation  SourceProductBaseCode=VR
  Azimuth : Outport
  Elevation : Outport  Port=2
  z : Outport  Port=3
  wires:
  MATLAB Function8/1(azimuth_rad) -> Azimuth/1
  MATLAB Function9/1(elevation) -> Elevation/1
  Normalize Vector17/1 -> MATLAB Function8/1(vec), MATLAB Function9/1(vec)
  Sun_B/1 -> Normalize Vector17/1
  MATLAB Function9/2(z) -> z/1

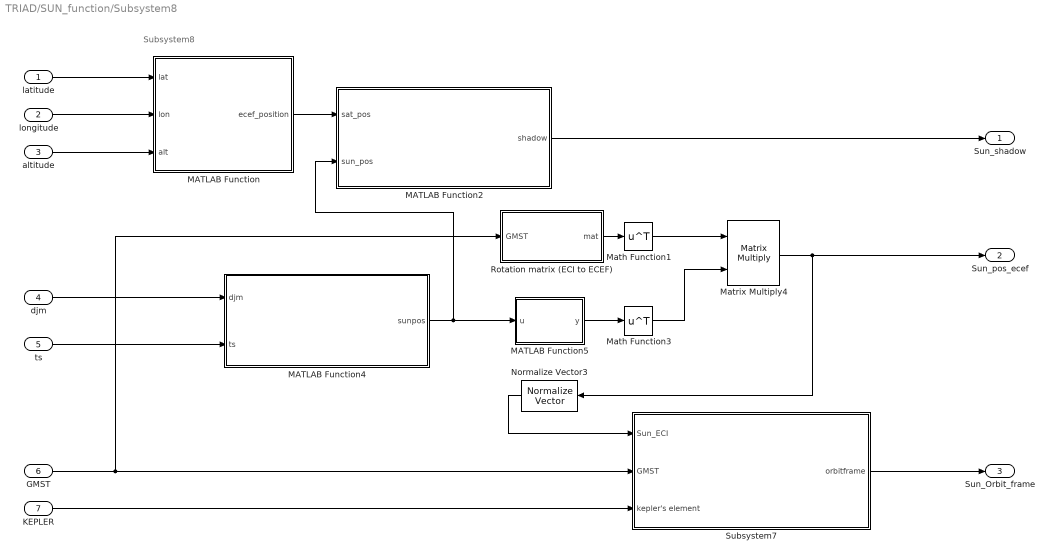
== system TRIAD/SUN_function/Subsystem8 ==
  note: Subsystem8
  latitude : Inport
  longitude : Inport  Port=2
  altitude : Inport  Port=3
  djm : Inport  Port=4
  ts : Inport  Port=5
  GMST : Inport  Port=6
  KEPLER : Inport  Port=7
  MATLAB Function : MATLAB Function  TreatAsAtomicUnit=on
  MATLAB Function2 : MATLAB Function  TreatAsAtomicUnit=on
  MATLAB Function4 : MATLAB Function  TreatAsAtomicUnit=on
  MATLAB Function5 : MATLAB Function  TreatAsAtomicUnit=on
  Math Function1 : Math  Operator=transpose  SaturateOnIntegerOverflow=on
  Math Function3 : Math  Operator=transpose  SaturateOnIntegerOverflow=on
  Matrix Multiply4 : Product  Multiplication=Matrix(*)
  Normalize Vector3 : vrlib/Utilities/Normalize Vector  maxzero=0
      settings: SourceProductName=Simulink 3D Animation  SourceProductBaseCode=VR
  Rotation matrix (ECI to ECEF) : MATLAB Function  TreatAsAtomicUnit=on
  Subsystem7 : Subsystem
  Sun_shadow : Outport
  Sun_pos_ecef : Outport  Port=2
  Sun_Orbit_frame : Outport  Port=3
  wires:
  ts/1 -> MATLAB Function4/2(ts)
  djm/1 -> MATLAB Function4/1(djm)
  KEPLER/1 -> Subsystem7/3(kepler's element)
  Subsystem7/1(orbitframe) -> Sun_Orbit_frame/1
  MATLAB Function4/1(sunpos) -> MATLAB Function5/1(u), MATLAB Function2/2(sun_pos)
  longitude/1 -> MATLAB Function/2(lon)
  MATLAB Function2/1(shadow) -> Sun_shadow/1
  latitude/1 -> MATLAB Function/1(lat)
  MATLAB Function/1(ecef_position) -> MATLAB Function2/1(sat_pos)
  altitude/1 -> MATLAB Function/3(alt)
  Rotation matrix (ECI to ECEF)/1(mat) -> Math Function1/1
  MATLAB Function5/1(y) -> Math Function3/1
  Math Function3/1 -> Matrix Multiply4/2
  Matrix Multiply4/1 -> Normalize Vector3/1, Sun_pos_ecef/1
  Math Function1/1 -> Matrix Multiply4/1
  GMST/1 -> Rotation matrix (ECI to ECEF)/1(GMST), Subsystem7/2(GMST)
  Normalize Vector3/1 -> Subsystem7/1(Sun_ECI)

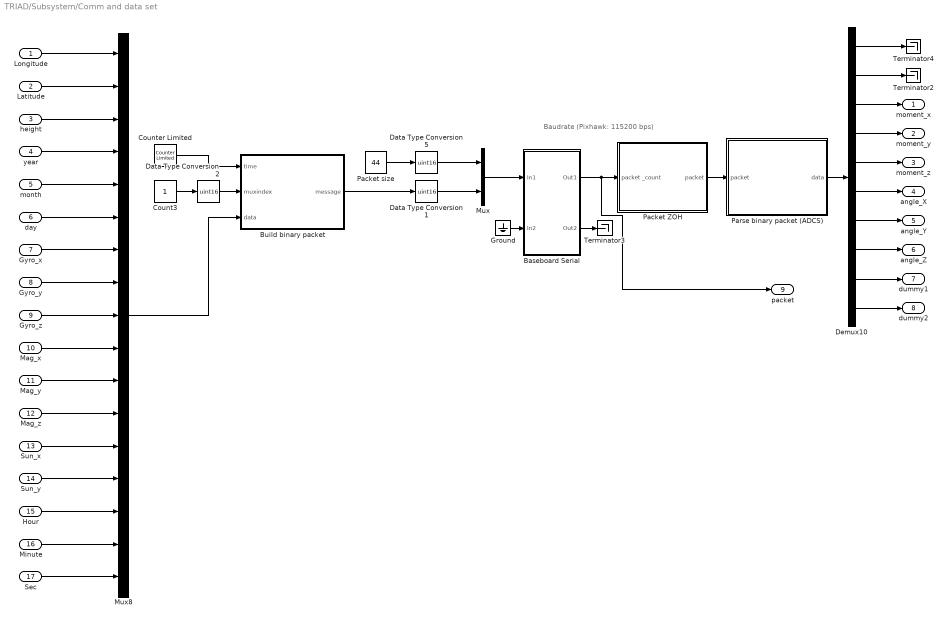
== system TRIAD/Subsystem/Comm and data set ==
  note: Baudrate (Pixhawk: 115200 bps)
  Longitude : Inport
  Latitude : Inport  Port=2
  height : Inport  Port=3
  year : Inport  Port=4
  month : Inport  Port=5
  day : Inport  Port=6
  Gyro_x : Inport  Port=7
  Gyro_y : Inport  Port=8
  Gyro_z : Inport  Port=9
  Mag_x : Inport  Port=10
  Mag_y : Inport  Port=11
  Mag_z : Inport  Port=12
  Sun_x : Inport  Port=13
  Sun_y : Inport  Port=14
  Hour : Inport  Port=15
  Minute : Inport  Port=16
  Sec : Inport  Port=17
  Baseboard Serial : Subsystem  InitFcn=mbaseserialmask(4,2);  mask(Baseboard RS232 Send Receive){group=Receive Setup, port=1, irqnum=4, saddr1=0x3f8, saddr2=0x3e8, config=Com1/none, baud1=115200, parity1=None, ndata1=8, nstop1=1, fifomode1=64 deep, rlevel1=half full, automode1=off, xmtfifosize1=1024, xmtdatatype1=count+16 bit uint, rcvfifosize1=1024, rcvmaxread1=22, rcvminread1=1, rcvusedelim1=off, rcvdelim1=13, rcvdatatype1=count+16 bit uint, rcvsampletime1=0.05, baud2=115200, parity2=None, ndata2=8, nstop2=1, fifomode2=16 deep, rlevel2=half full, automode2=off, xmtfifosize2=1024, xmtdatatype2=count+16 bit uint, rcvfifosize2=1024, rcvmaxread2=1024, rcvminread2=1, rcvusedelim2=on, rcvdelim2=13, rcvdatatype2=count+16 bit uint, rcvsampletime2=0.1}
      mask prompts: group "Parameter group:"; port "Port to modify:"; irqnum "IRQ number:"; saddr1 "First port address:"; saddr2 "Second port address:"; config "Configuration:"; baud1 "Baud rate:"; parity1 "Parity:"; ndata1 "Data bits:"; nstop1 "Stop bits:"; fifomode1 "Hardware FIFO size:"; rlevel1 "Receive FIFO interrupt level:"; automode1 "Auto RTS/CTS:"; xmtfifosize1 "Transmit software FIFO size:"; xmtdatatype1 "Transmit FIFO data type:"; rcvfifosize1 "Receive software FIFO size:"; rcvmaxread1 "Receive maximum read:"; rcvminread1 "Receive minimum read:"; rcvusedelim1 "Read to delimiter:"; rcvdelim1 "Delimiter:"; rcvdatatype1 "Receive data type:"; rcvsampletime1 "Receive SampleTime:"; baud2 "Baud rate:"; parity2 "Parity:"; ndata2 "Data bits:"; nstop2 "Stop bits:"; fifomode2 "Hardware FIFO size:"; rlevel2 "Receive FIFO interrupt level:"; automode2 "Auto RTS/CTS:"; xmtfifosize2 "Transmit software FIFO size:"; xmtdatatype2 "Transmit FIFO data type:"; rcvfifosize2 "Receive software fifo size:"; rcvmaxread2 "Receive maximum read:"; rcvminread2 "Receive minimum read:"; rcvusedelim2 "Read to delimiter:"; rcvdelim2 "Delimiter:"; rcvdatatype2 "Receive data type:"; rcvsampletime2 "Receive SampleTime:"
      mask help:
      | Baseboard
      | RS232 Send Receive Subsystem
      mask init:
      | [addr1, addr2, maskdisplay] = mbaseserialmask( 1, 2 );
      | baddr1 = addr1;
      | baddr2 = addr2;
      | mbaseserialmask( 3, 2 );
      | set_param( gcb, 'MaskDisplay', maskdisplay );
      mask Help: eval('xpcdoc(''Baseboard_Serial_Subsystem'')');
      mask TypeOptions group: Board Setup | Basic Setup | Transmit Setup | Receive Setup
      mask Callback group: mbaseserialmask( 2, 2 );
      mask TypeOptions port: 1 | 2
      mask Callback port: mbaseserialmask( 2, 2 );
      mask TypeOptions config: Com1/none | Com2/none | Com1/Com3 | Com2/Com4 | none/Com3 | none/Com4 | Custom
      mask Callback config: mbaseserialmask( 2, 2 );
      mask TypeOptions baud1: 115200 | 57600 | 38400 | 19200 | 9600 | 4800 | 2400 | 1200 | 600 | 300 | 110
      mask TypeOptions parity1: None | Even | Odd | Mark | Space
      mask TypeOptions ndata1: 5 | 6 | 7 | 8
      mask TypeOptions nstop1: 1 | 2
      mask TypeOptions fifomode1: 64 deep | 16 deep | 1 deep
      mask TypeOptions rlevel1: 1 | quarter full | half full | almost full
      mask TypeOptions xmtdatatype1: count+32 bit int | count+32 bit uint | count+16 bit int | count+16 bit uint | 8 bit int null terminated | 8 bit uint null terminated
      mask TypeOptions rcvdatatype1: count+32 bit int | count+32 bit uint | count+16 bit int | count+16 bit uint | 8 bit int null terminated | 8 bit uint null terminated
      mask TypeOptions baud2: 115200 | 57600 | 38400 | 19200 | 9600 | 4800 | 2400 | 1200 | 600 | 300 | 110
      mask TypeOptions parity2: None | Even | Odd | Mark | Space
      mask TypeOptions ndata2: 5 | 6 | 7 | 8
      mask TypeOptions nstop2: 1 | 2
      mask TypeOptions fifomode2: 64 deep | 16 deep | 1 deep
      mask TypeOptions rlevel2: 1 | quarter full | half full | almost full
      mask TypeOptions xmtdatatype2: count+32 bit int | count+32 bit uint | count+16 bit int | count+16 bit uint | 8 bit int null terminated | 8 bit uint null terminated
      mask TypeOptions rcvdatatype2: count+32 bit int | count+32 bit uint | count+16 bit int | count+16 bit uint | 8 bit int null terminated | 8 bit uint null terminated
      mask Display: disp('Baseboard\nRS232\nSend Receive');port_label('input',1,'XMT1');port_label('input',2,'');port_label('output',1,'RCV1');port_label('output',2,'');
  Build binary packet : MATLAB Function  TreatAsAtomicUnit=on
  Count3 : Constant  SampleTime=-1
  Counter Limited : simulink/Sources/Counter Limited  uplimit=1000000  tsamp=-1
  Data Type Conversion1 : DataTypeConversion  OutDataTypeStr=uint16
  Data Type Conversion2 : DataTypeConversion  OutDataTypeStr=uint16
  Data Type Conversion5 : DataTypeConversion  OutDataTypeStr=uint16
  Demux10 : Demux  Outputs=10
  Ground : Ground
  Mux : Mux  Inputs=2
  Mux8 : Mux  Inputs=17
  Packet ZOH : Subsystem
  Packet size : Constant  Value=44  SampleTime=-1
  Parse binary packet (ADCS) : MATLAB Function  TreatAsAtomicUnit=on
  Terminator2 : Terminator
  Terminator3 : Terminator
  Terminator4 : Terminator
  moment_x : Outport
  moment_y : Outport  Port=2
  moment_z : Outport  Port=3
  angle_X : Outport  Port=4
  angle_Y : Outport  Port=5
  angle_Z : Outport  Port=6
  dummy1 : Outport  Port=7
  dummy2 : Outport  Port=8
  packet : Outport  Port=9
  wires:
  Demux10/6 -> angle_X/1
  Data Type Conversion5/1 -> Mux/1
  Count3/1 -> Data Type Conversion2/1
  Parse binary packet (ADCS)/1(data) -> Demux10/1
  Demux10/5 -> moment_z/1
  Demux10/2 -> Terminator2/1
  Baseboard Serial/1(Out1) -> packet/1, Packet ZOH/1(packet _count)
  Packet size/1 -> Data Type Conversion5/1
  Data Type Conversion1/1 -> Mux/2
  Longitude/1 -> Mux8/1
  Demux10/4 -> moment_y/1
  Packet ZOH/1(packet) -> Parse binary packet (ADCS)/1(packet)
  Build binary packet/1(message) -> Data Type Conversion1/1
  Demux10/1 -> Terminator4/1
  Counter Limited/1 -> Build binary packet/1(time)
  Latitude/1 -> Mux8/2
  Demux10/3 -> moment_x/1
  height/1 -> Mux8/3
  Mux/1 -> Baseboard Serial/1(In1)
  Data Type Conversion2/1 -> Build binary packet/2(muxindex)
  Mux8/1 -> Build binary packet/3(data)
  Baseboard Serial/2(Out2) -> Terminator3/1
  Ground/1 -> Baseboard Serial/2(In2)
  Sun_y/1 -> Mux8/14
  Sun_x/1 -> Mux8/13
  Mag_z/1 -> Mux8/12
  Mag_y/1 -> Mux8/11
  Mag_x/1 -> Mux8/10
  Gyro_z/1 -> Mux8/9
  Gyro_y/1 -> Mux8/8
  Gyro_x/1 -> Mux8/7
  year/1 -> Mux8/4
  month/1 -> Mux8/5
  day/1 -> Mux8/6
  Demux10/7 -> angle_Y/1
  Demux10/8 -> angle_Z/1
  Demux10/9 -> dummy1/1
  Demux10/10 -> dummy2/1
  Hour/1 -> Mux8/15
  Minute/1 -> Mux8/16
  Sec/1 -> Mux8/17

== system TRIAD/Subsystem10/Subsystem7 ==
  torque : Inport
  init_gyro : Inport  Port=2
  eular rotational equation2 : Subsystem
  innertial momoent1 : Constant  Value=[0.03889 0 0 ; 0 0.03184 0 ;0 0 0.03908]
  omega : Outport
  omega_dot : Outport  Port=2
  wires:
  eular rotational equation2/1(omega) -> omega/1
  init_gyro/1 -> eular rotational equation2/3(omega_0)
  torque/1 -> eular rotational equation2/1(Torque)
  innertial momoent1/1 -> eular rotational equation2/2(Inertial)
  eular rotational equation2/2(omega_dot) -> omega_dot/1

== system TRIAD/Subsystem10/Subsystem8 ==
  init_quat : Inport
  omega : Inport  Port=2
  Integrator2 : Integrator  InitialConditionSource=external
  Kinematics (quaternion2)1 : Subsystem  mask(Kinematics: quat2){}
      mask help:
      | q0 = cos(phi/2)
      | q1 = e1*sin(phi/2)
      | q2 = e2*sin(phi/2)
      | q3 = e3*sin(phi/2)
  quat to Euler1 : Subsystem  mask(quat2_to_Euler){}
      mask help:
      | % Input: Quaternion Definition
      | q0 = cos(phi/2)
      | q1 = e1*sin(phi/2)
      | q2 = e2*sin(phi/2)
      | q3 = e3*sin(phi/2)
      | where, phi: Eigenaxis rotation angle, [e1 e2 e3]: Eigenaxis rotation vector
      |
      | % Output: 3(Psi)-2(Theta)-1(Phi) Euler angle
  v_2 : dspmathops/Normalization  NormType=2-norm  Bias=1e-10  NormOver=Each row  Dimension=1  outputDataTypeStr=Inherit: Same as product output  outputLastDataTypeStr=Inherit: Same as product output  outputMin=[]  outputMax=[]  accumDataTypeStr=Inherit: Same as product output  accumLastDataTypeStr=Inherit: Same as product output  roundingMode=Floor  overflowMode=off
      settings: SourceProductName=DSP System Toolbox
  quaternion : Outport
  euler : Outport  Port=2
  wires:
  Integrator2/1 -> quat to Euler1/1(quat), v_2/1
  v_2/1 -> quaternion/1, Kinematics (quaternion2)1/1(quat)
  Kinematics (quaternion2)1/1(quat2dot) -> Integrator2/1
  init_quat/1 -> Integrator2/2
  omega/1 -> Kinematics (quaternion2)1/2(omega)
  quat to Euler1/1(euler) -> euler/1

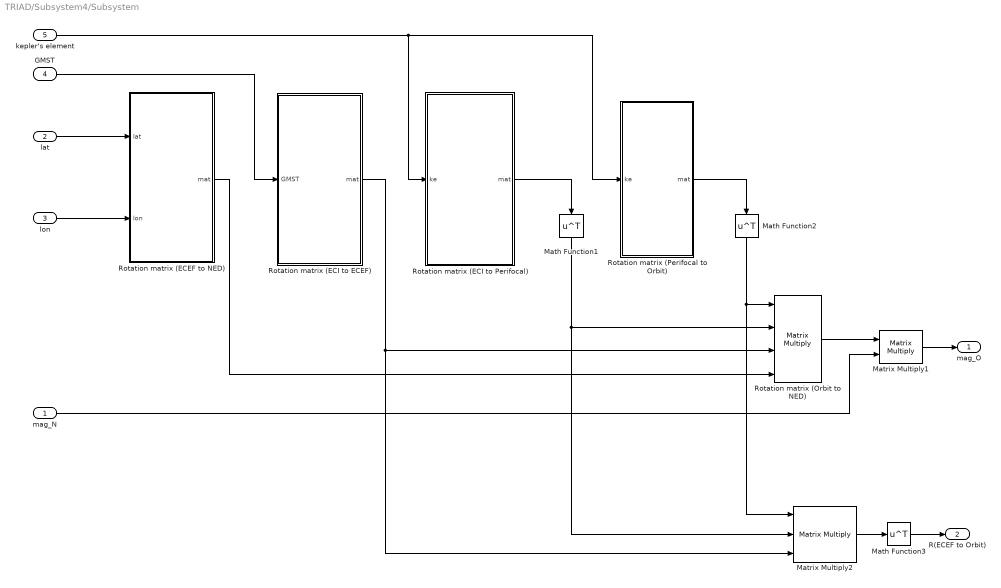
== system TRIAD/Subsystem4/Subsystem ==
  mag_N : Inport
  lat : Inport  Port=2
  lon : Inport  Port=3
  GMST : Inport  Port=4
  kepler's element : Inport  Port=5
  Math Function1 : Math  Operator=transpose  SaturateOnIntegerOverflow=on
  Math Function2 : Math  Operator=transpose  SaturateOnIntegerOverflow=on
  Math Function3 : Math  Operator=transpose  SaturateOnIntegerOverflow=on
  Matrix Multiply1 : Product  Multiplication=Matrix(*)
  Matrix Multiply2 : Product  Inputs=3  Multiplication=Matrix(*)
  Rotation matrix (ECEF to NED) : MATLAB Function  TreatAsAtomicUnit=on
  Rotation matrix (ECI to ECEF) : MATLAB Function  TreatAsAtomicUnit=on
  Rotation matrix (Orbit to NED) : Product  Inputs=4  Multiplication=Matrix(*)
  Rotation matrix (ECI to Perifocal) : MATLAB Function  TreatAsAtomicUnit=on
  Rotation matrix (Perifocal to Orbit) : MATLAB Function  TreatAsAtomicUnit=on
  mag_O : Outport
  R(ECEF to Orbit) : Outport  Port=2
  wires:
  lat/1 -> Rotation matrix (ECEF to NED)/1(lat)
  lon/1 -> Rotation matrix (ECEF to NED)/2(lon)
  kepler's element/1 -> Rotation matrix (ECI to Perifocal)/1(ke), Rotation matrix (Perifocal to Orbit)/1(ke)
  Rotation matrix (Perifocal to Orbit)/1(mat) -> Math Function2/1
  Math Function2/1 -> Matrix Multiply2/1, Rotation matrix (Orbit to NED)/1
  GMST/1 -> Rotation matrix (ECI to ECEF)/1(GMST)
  Rotation matrix (ECI to Perifocal)/1(mat) -> Math Function1/1
  Math Function1/1 -> Matrix Multiply2/2, Rotation matrix (Orbit to NED)/2
  Rotation matrix (ECI to ECEF)/1(mat) -> Matrix Multiply2/3, Rotation matrix (Orbit to NED)/3
  Rotation matrix (ECEF to NED)/1(mat) -> Rotation matrix (Orbit to NED)/4
  Rotation matrix (Orbit to NED)/1 -> Matrix Multiply1/1
  mag_N/1 -> Matrix Multiply1/2
  Matrix Multiply1/1 -> mag_O/1
  Matrix Multiply2/1 -> Math Function3/1
  Math Function3/1 -> R(ECEF to Orbit)/1

== system TRIAD/Subsystem9/Subsystem7 ==
  torque : Inport
  init_gyro : Inport  Port=2
  eular rotational equation2 : Subsystem
  innertial momoent1 : Constant  Value=[0.03889 0 0 ; 0 0.03184 0 ;0 0 0.03908]
  omega : Outport
  omega_dot : Outport  Port=2
  wires:
  eular rotational equation2/1(omega) -> omega/1
  init_gyro/1 -> eular rotational equation2/3(omega_0)
  torque/1 -> eular rotational equation2/1(Torque)
  innertial momoent1/1 -> eular rotational equation2/2(Inertial)
  eular rotational equation2/2(omega_dot) -> omega_dot/1

== system TRIAD/Subsystem9/Subsystem8 ==
  init_quat : Inport
  omega : Inport  Port=2
  Gain11 : Gain  Gain=(180)/pi
  Integrator2 : Integrator  InitialConditionSource=external
  Kinematics (quaternion2)1 : Subsystem  mask(Kinematics: quat2){}
      mask help:
      | q0 = cos(phi/2)
      | q1 = e1*sin(phi/2)
      | q2 = e2*sin(phi/2)
      | q3 = e3*sin(phi/2)
  quat to Euler1 : Subsystem  mask(quat2_to_Euler){}
      mask help:
      | % Input: Quaternion Definition
      | q0 = cos(phi/2)
      | q1 = e1*sin(phi/2)
      | q2 = e2*sin(phi/2)
      | q3 = e3*sin(phi/2)
      | where, phi: Eigenaxis rotation angle, [e1 e2 e3]: Eigenaxis rotation vector
      |
      | % Output: 3(Psi)-2(Theta)-1(Phi) Euler angle
  v_2 : dspmathops/Normalization  NormType=2-norm  Bias=1e-10  NormOver=Each row  Dimension=1  outputDataTypeStr=Inherit: Same as product output  outputLastDataTypeStr=Inherit: Same as product output  outputMin=[]  outputMax=[]  accumDataTypeStr=Inherit: Same as product output  accumLastDataTypeStr=Inherit: Same as product output  roundingMode=Floor  overflowMode=off
      settings: SourceProductName=DSP System Toolbox
  quaternion : Outport
  euler : Outport  Port=2
  wires:
  Integrator2/1 -> quat to Euler1/1(quat), v_2/1
  v_2/1 -> quaternion/1, Kinematics (quaternion2)1/1(quat)
  Kinematics (quaternion2)1/1(quat2dot) -> Integrator2/1
  init_quat/1 -> Integrator2/2
  omega/1 -> Kinematics (quaternion2)1/2(omega)
  quat to Euler1/1(euler) -> Gain11/1
  Gain11/1 -> euler/1

== system TRIAD/SUN_function/Subsystem8/Subsystem7 ==
  Sun_ECI : Inport
  GMST : Inport  Port=2
  kepler's element : Inport  Port=3
  Math Function1 : Math  Operator=transpose  SaturateOnIntegerOverflow=on
  Math Function2 : Math  Operator=transpose  SaturateOnIntegerOverflow=on
  Math Function4 : Math  Operator=transpose  SaturateOnIntegerOverflow=on
  Matrix Multiply1 : Product  Multiplication=Matrix(*)
  Matrix Multiply2 : Product  Multiplication=Matrix(*)
  Matrix Multiply3 : Product  Multiplication=Matrix(*)
  Matrix Multiply4 : Product  Inputs=3  Multiplication=Matrix(*)
  Rotation matrix (ECI to ECEF) : MATLAB Function  TreatAsAtomicUnit=on
  Rotation matrix (ECI to Perifocal) : MATLAB Function  TreatAsAtomicUnit=on
  Rotation matrix (Perifocal to Orbit) : MATLAB Function  TreatAsAtomicUnit=on
  orbitframe : Outport
  wires:
  GMST/1 -> Rotation matrix (ECI to ECEF)/1(GMST)
  Matrix Multiply2/1 -> Math Function4/1
  Math Function4/1 -> Matrix Multiply1/1
  Matrix Multiply4/1 -> Matrix Multiply3/1
  Sun_ECI/1 -> Matrix Multiply3/2
  Matrix Multiply3/1 -> orbitframe/1
  Rotation matrix (ECI to ECEF)/1(mat) -> Matrix Multiply4/3
  kepler's element/1 -> Rotation matrix (Perifocal to Orbit)/1(ke), Rotation matrix (ECI to Perifocal)/1(ke)
  Rotation matrix (ECI to Perifocal)/1(mat) -> Math Function1/1
  Rotation matrix (Perifocal to Orbit)/1(mat) -> Math Function2/1
  Math Function1/1 -> Matrix Multiply4/2
  Math Function2/1 -> Matrix Multiply4/1

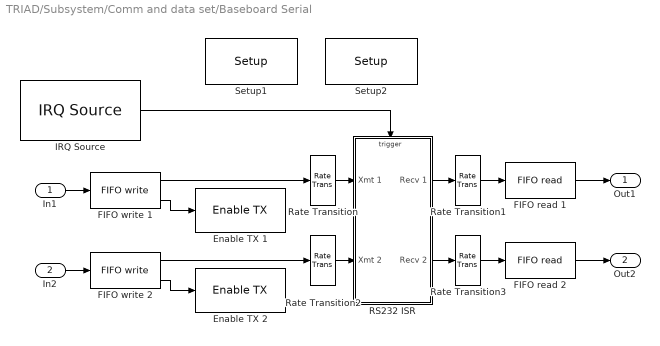
== system TRIAD/Subsystem/Comm and data set/Baseboard Serial ==
  In1 : Inport
  In2 : Inport  Port=2
  Enable TX 1 : xpcseriallib/Mainboard/Baseboard Serial Internal  blocks/Enable TX   addr=baddr1
      settings: SourceProductName=Simulink Real-Time  SourceProductBaseCode=XP
  Enable TX 2 : xpcseriallib/Mainboard/Baseboard Serial Internal  blocks/Enable TX   addr=baddr2
      settings: SourceProductName=Simulink Real-Time  SourceProductBaseCode=XP
  FIFO read 1 : xpcseriallib/FIFO read   maxsize=22  minsize=1  usedelimiter=off  delimiter=13  outputtype=count+16 bit uint  enable=off  enableout=off  sampletime=0.05
      settings: SourceProductName=Simulink Real-Time  SourceProductBaseCode=XP
  FIFO read 2 : xpcseriallib/FIFO read   maxsize=1024  minsize=1  usedelimiter=on  delimiter=13  outputtype=count+16 bit uint  enable=off  enableout=off  sampletime=0.1
      settings: SourceProductName=Simulink Real-Time  SourceProductBaseCode=XP
  FIFO write 1 : xpcseriallib/FIFO write   size=1024  inputtype=count+16 bit uint  present=on  sampletime=0.05  id=XMT channel 1, IRQ 4
      settings: SourceProductName=Simulink Real-Time  SourceProductBaseCode=XP
  FIFO write 2 : xpcseriallib/FIFO write   size=1024  inputtype=count+16 bit uint  present=on  sampletime=0.05  id=XMT channel 2, IRQ 4
      settings: SourceProductName=Simulink Real-Time  SourceProductBaseCode=XP
  IRQ Source : slrtlib/Asynchronous Event/IRQ Source   irqNo=4  preempt=10  b_type=None/Other  slot=-1  isrPrio=0
      settings: SourceProductName=Simulink Real-Time  SourceProductBaseCode=XP
  RS232 ISR : Subsystem  TreatAsAtomicUnit=on  mask(RS232 ISR){addr1=baddr1, addr2=baddr2}
      mask prompts: addr1 "First channel address:"; addr2 "Second channel address:"
      mask help:
      | Baseboard Serial
      | Interrupt Service Routine
      mask init:
      | baddr1 = addr1;
      | baddr2 = addr2;
      mask Display:
      | disp('Baseboard\nSerial\nISR');
      | port_label('input', 1, 'XMT1');
      | port_label('input', 2, 'XMT3');
      | port_label('output', 1, 'RCV1');
      | port_label('output', 2, 'RCV3');
  Rate Transition{,1..3} (4 alike) : RateTransition  Integrity=off  Deterministic=off
  Setup1 : xpcseriallib/Mainboard/Baseboard Serial Internal  blocks/Setup  baud=115200  width=8  nstop=1  parity=None  fmode=64 deep  rlevel=half full  ctsmode=off  addr=baddr1
      settings: SourceProductName=Simulink Real-Time  SourceProductBaseCode=XP
  Setup2 : xpcseriallib/Mainboard/Baseboard Serial Internal  blocks/Setup  baud=115200  width=8  nstop=1  parity=None  fmode=16 deep  rlevel=half full  ctsmode=off  addr=baddr2
      settings: SourceProductName=Simulink Real-Time  SourceProductBaseCode=XP
  Out1 : Outport
  Out2 : Outport  Port=2
  wires:
  FIFO write 1/2 -> Enable TX 1/1
  IRQ Source/1 -> RS232 ISR/Trigger
  FIFO write 1/1 -> Rate Transition/1
  In1/1 -> FIFO write 1/1
  FIFO write 2/1 -> Rate Transition2/1
  In2/1 -> FIFO write 2/1
  Rate Transition1/1 -> FIFO read 1/1
  FIFO read 1/1 -> Out1/1
  Rate Transition3/1 -> FIFO read 2/1
  FIFO read 2/1 -> Out2/1
  FIFO write 2/2 -> Enable TX 2/1
  Rate Transition2/1 -> RS232 ISR/2(Xmt 2)
  Rate Transition/1 -> RS232 ISR/1(Xmt 1)
  RS232 ISR/1(Recv 1) -> Rate Transition1/1
  RS232 ISR/2(Recv 2) -> Rate Transition3/1
